simulink model "Project1LibVer"  (R2017b)
settings: Solver=FixedStepAuto  StartTime=0.0  StopTime=inf  RelTol=1e-3
libraries: RoombaSimulink x3, realtime_pacer_lib x1, simulink x1
settings Model: Creator=Mark  LastModifiedBy=Mark

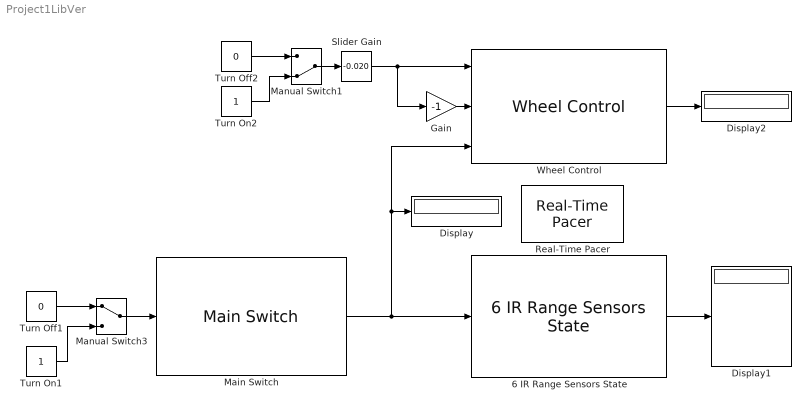
== system Project1LibVer ==
  6 IR Range Sensors State : RoombaSimulink/6 IR Range Sensors State
  Display : Display
  Display1 : Display
  Display2 : Display
  Gain : Gain  Gain=-1
  Main Switch : RoombaSimulink/Main Switch
  Manual Switch1 : ManualSwitch  CurrentSetting=0
  Manual Switch3 : ManualSwitch
  Real-Time Pacer : realtime_pacer_lib/Real-Time Pacer  simTimePerRealTime=1
  Slider Gain : simulink/Math Operations/Slider Gain  gain=-0.020  low=-0.5  high=0.5
  Turn Off1 : Constant  Value=0
  Turn Off2 : Constant  Value=0
  Turn On1 : Constant
  Turn On2 : Constant
  Wheel Control : RoombaSimulink/Wheel Control
  wires:
  Main Switch/1 -> Display/1, Wheel Control/3, 6 IR Range Sensors State/1
  Turn On1/1 -> Manual Switch3/2
  Turn Off1/1 -> Manual Switch3/1
  Manual Switch3/1 -> Main Switch/1
  Gain/1 -> Wheel Control/2
  Slider Gain/1 -> Wheel Control/1, Gain/1
  Turn On2/1 -> Manual Switch1/2
  Turn Off2/1 -> Manual Switch1/1
  6 IR Range Sensors State/1 -> Display1/1
  Wheel Control/1 -> Display2/1
  Manual Switch1/1 -> Slider Gain/1
